simulink model "Task1"  (R2023a)
settings: Solver=VariableStepAuto  StartTime=0.0  StopTime=8  RelTol=1e-3
libraries: cstblocks x4
settings Model: Creator=MUHAMMAD SADEEQ  LastModifiedBy=MUHAMMAD SADEEQ

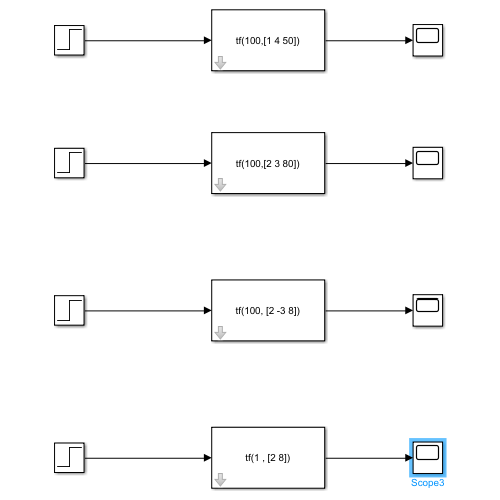
[thumbnail: Simulink's stored preview of the top-level diagram]
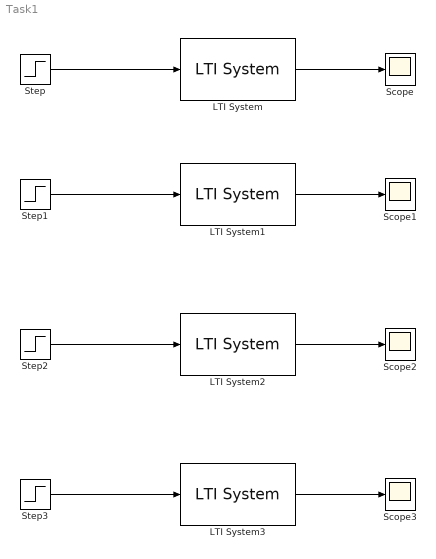
== system Task1 ==
  LTI System : cstblocks/LTI System  sys=tf(100,[1 4 50])  IC=[]
  LTI System1 : cstblocks/LTI System  sys=tf(100,[2 3 80])  IC=[]
  LTI System2 : cstblocks/LTI System  sys=tf(100, [2 -3 8])  IC=[]
  LTI System3 : cstblocks/LTI System  sys=tf(1 , [2 8])  IC=[]
  Scope{,1..3} (4 alike) : Scope
  Step{,1..3} (4 alike) : Step  SampleTime=0
  wires:
  LTI System/1 -> Scope/1
  Step/1 -> LTI System/1
  LTI System1/1 -> Scope1/1
  Step1/1 -> LTI System1/1
  Step2/1 -> LTI System2/1
  LTI System2/1 -> Scope2/1
  LTI System3/1 -> Scope3/1
  Step3/1 -> LTI System3/1
